simulink model "simulation_staticParameters"  (R2016b)
settings: Solver=VariableStepAuto  StartTime=0.0  StopTime=10  RelTol=1e-3
settings Model: Creator=user  LastModifiedBy=user

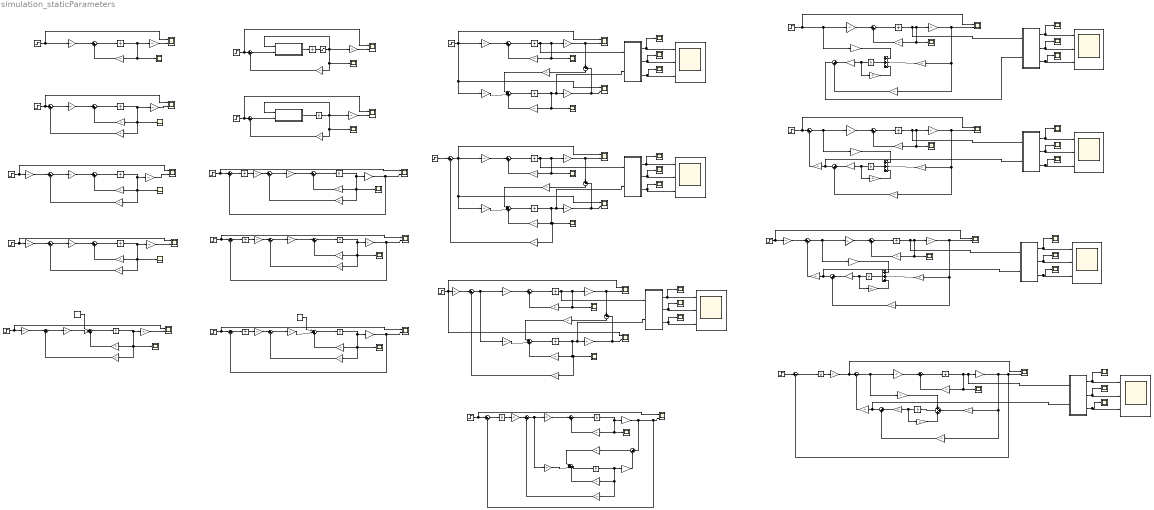
== system simulation_staticParameters ==
  note: FULL ORDER OBSERVER
  note: e_dot
  note: e
  note: y
  note: STATE FEEDBACK APPLIED
  note: NO STATE FEEDBACK
  note: input
  note: y
  note: x
  note: x_dot
  note: input
  note: y
  note: x
  note: x_dot
  note: STATE FEEDBACK + STATIC PRE-FILTER APPLIED
  note: input
  note: y
  note: x
  note: x_dot
  note: STATE FEEDBACK + STATIC PRE-FILTER APPLIED: PARAMETER CHANGE
  note: input
  note: y
  note: x
  note: x_dot
  note: STATE FEEDBACK + STATIC PRE-FILTER APPLIED: CONST DISTURBANCE
  note: input
  note: y
  note: x
  note: x_dot
  note: STATE FEEDBACK APPLIED on NONLINEAR SYSTEM
  note: input
  note: y
  note: STATE FEEDBACK APPLIED on NONLINEAR SYSTEM: zero inititial conditions
  note: input
  note: y
  note: STATE FEEDBACK + DYNAMIC COMPENSATOR APPLIED
  note: input
  note: x
  note: x_dot
  note: y
  note: STATE FEEDBACK + DYNAMIC COMPENSATOR APPLIED : PARAMETER CHANGE
  note: input
  note: x
  note: x_dot
  note: STATE FEEDBACK + DYNAMIC COMPENSATOR APPLIED: CONST DISTURBANCE
  note: y
  note: input
  note: x
  note: x_dot
  note: input
  note: y
  note: x
  note: x_dot
  note: input
  note: y
  note: x
  note: x_dot
  note: STATE FEEDBACK USING FULL ORDER OBSERVER
  note: input
  note: y
  note: x
  note: x_dot
  note: input
  note: y
  note: x
  note: x_dot
  note: STATE FEEDBACK + STATIC PRE-FILTER USING FULL ORDER OBSERVER
  note: input
  note: y
  note: x
  note: x_dot
  note: input
  note: y
  note: x
  note: x_dot
  note: y
  note: STATE FEEDBACK + DYNAMIC COMPENSATOR USING FULL ORDER OBSERVER
  note: input
  note: x
  note: x_dot
  note: x
  note: x_dot
  note: x
  note: x_dot
  note: input
  note: y
  note: REDUCED ORDER OBSERVER
  note: x
  note: x_dot
  note: input
  note: y
  note: STATE FEEDBACK USING REDUCED ORDER OBSERVER
  note: x
  note: x_dot
  note: input
  note: y
  note: STATE FEEDBACK + STATIC PRE-FILTER USING REDUCED ORDER OBSERVER
  note: x
  note: x_dot
  note: input
  note: y
  note: STATE FEEDBACK + DYNAMIC COMPENSATOR USING REDUCED ORDER OBSERVER
  A{1..5,7..20} (19 alike) : Gain  Gain=[0,0.1963,0;-0.1963,0,0.9817;0,0,0]  Multiplication=Matrix(K*u)
  A6 : Gain  Gain=[0,0.1963,0;-0.1963,0,0.9817;0,0,0]*1.05  Multiplication=Matrix(K*u)
  B{,1..2,4,8..13} (10 alike) : Gain  Gain=[0.025, 0.025;0,0;-0.333, 0.333]  Multiplication=Matrix(K*u)
  B{5,7,14..15} (4 alike) : Gain  Gain=[0.025;0;-0.333]  Multiplication=Matrix(K*u)
  B3 : Gain  Gain=[0.025, 0.025;0,0;-0.333, 0.333]*1.2  Multiplication=Matrix(K*u)
  B6 : Gain  Gain=[0.025;0;-0.333]*1.1  Multiplication=Matrix(K*u)
  C{1..5,7,11..16,19..21} (15 alike) : Gain  Gain=[1,0,0;0,1,0]  Multiplication=Matrix(K*u)
  C{8,10,17..18} (4 alike) : Gain  Gain=[1,0,0;]  Multiplication=Matrix(K*u)
  C22 : Gain  Gain=[1,0,0]  Multiplication=Matrix(K*u)
  C6 : Gain  Gain=[1,0,0;0,1,0]*1.1  Multiplication=Matrix(K*u)
  C9 : Gain  Gain=[1,0,0;]*1.05  Multiplication=Matrix(K*u)
  Constant : Constant  Value=2
  Constant1 : Constant  Value=10
  D : Gain  Gain=-21
  D1 : Gain  Gain=-21
  D2 : Gain  Gain=-21
  D3 : Gain  Gain=[0 -470.63; 0.9817 -3.583]  Multiplication=Matrix(K*u)
  G^-1(0){,1..4} (5 alike) : Gain  Gain=[394.735, -188.5098; 406.3311, -94.8546]  Multiplication=Matrix(K*u)
  Gain1 : Gain  Gain=[-.308 .358]  Multiplication=Matrix(K*u)
  Gain2 : Gain  Gain=[-.308 .358]  Multiplication=Matrix(K*u)
  Gain3 : Gain  Gain=[388.4933, -184.5838, 31.2146; 395.0384, -90.9286, 56.4750]  Multiplication=Matrix(K*u)
  Gain4 : Gain  Gain=[388.4933, -184.5838, 31.2146; 395.0384, -90.9286, 56.4750]  Multiplication=Matrix(K*u)
  Gain5 : Gain  Gain=[-60.270750000000010;-0.456600000000000]  Multiplication=Matrix(K*u)
  Gain6 : Gain  Gain=[-71699, -18130, -5530]  Multiplication=Matrix(K*u)
  Integrator{,1..4,6..7,9,11,17..19,21} (13 alike) : Integrator  InitialCondition=[0,0,0]
  Integrator{8,10,12,20,30} (5 alike) : Integrator  InitialCondition=[0]
  Integrator{13,15,22,24,26,28} (6 alike) : Integrator  InitialCondition=[1,2,3]
  Integrator14 : Integrator  InitialCondition=[2,4,10]
  Integrator16 : Integrator  InitialCondition=[2,4,5]
  Integrator23 : Integrator  InitialCondition=4
  Integrator25 : Integrator  InitialCondition=4
  Integrator27 : Integrator
  Integrator29 : Integrator  InitialCondition=[4,5]
  Integrator5 : Integrator  InitialCondition=[0.05,0.01,0.1]
  K{,1..2,9..10,12} (6 alike) : Gain  Gain=[388.4933, -184.5838, 31.2146; 395.0384, -90.9286, 56.4750]  Multiplication=Matrix(K*u)
  K{6..8,11} (4 alike) : Gain  Gain=[-71699, -18130, -5530]  Multiplication=Matrix(K*u)
  K3 : Gain  Gain=[-2.324, -31.3649, -8.468; 19.532, -5.9637, 2.3224]  Multiplication=Matrix(K*u)
  K5 : Gain  Gain=[-2.324, -31.3649, -8.468; 19.532, -5.9637, 2.3224]  Multiplication=Matrix(K*u)
  Ki{,1..4} (5 alike) : Gain  Gain=[-209440]  Multiplication=Matrix(K*u)
  L : Gain  Gain=[21.998, 0.1916; -1.8526, 44.002; -37.5542, 492.0554]  Multiplication=Matrix(K*u)
  L1 : Gain  Gain=[21.998, 0.1916; -1.8526, 44.002; -37.5542, 492.0554]  Multiplication=Matrix(K*u)
  L2 : Gain  Gain=[21.998, 0.1916; -1.8526, 44.002; -37.5542, 492.0554]  Multiplication=Matrix(K*u)
  L3 : Gain  Gain=[66;7392;55141]  Multiplication=Matrix(K*u)
  MATLAB Function1 : MATLAB Function  TreatAsAtomicUnit=on
  MATLAB Function2 : MATLAB Function  TreatAsAtomicUnit=on
  MATLAB Function3 : MATLAB Function  TreatAsAtomicUnit=on
  MATLAB Function4 : MATLAB Function  TreatAsAtomicUnit=on
  MATLAB Function5 : MATLAB Function  TreatAsAtomicUnit=on
  MATLAB Function6 : MATLAB Function  TreatAsAtomicUnit=on
  MATLAB Function7 : MATLAB Function  TreatAsAtomicUnit=on
  R : Gain  Gain=[-.308 .358]  Multiplication=Matrix(K*u)
  Saturation : Saturate  UpperLimit=20  LowerLimit=-20
  Scope{,2,4,6,8,10,12..13,15,17,19,21,23,25,27,29,31,33,36,38,40} (21 alike) : Scope  NumInputPorts=2
  Scope{1,3,5,7,9,11,14,16,18,20,22,24,26,28,30,32,34..35,37,39,41} (21 alike) : Scope
  Step{1..7} (7 alike) : Step  Time=[2,4]  Before=[0,0]  After=[1,-.3]  SampleTime=0
  Step{8..10,14} (4 alike) : Step  Time=[2]  Before=[0]  After=[1]  SampleTime=0
  Step11 : Step  Time=[2,3]  Before=[1,1.5]  After=[2,2.5]  SampleTime=0
  Step12 : Step  Time=[2,3]  Before=[1,1.5]  After=[2,2.5]  SampleTime=0
  Step13 : Step  Time=[2,4]  Before=[0.5,-0.5]  After=[1,-.2]  SampleTime=0
  Step15 : Step  Time=[2,3]  Before=[0.5,1]  After=[1,2]  SampleTime=0
  Step16 : Step  Time=[2,3]  Before=[0.5,1]  After=[1,2]  SampleTime=0
  Step17 : Step  Time=[2,3]  Before=[0.5,1]  After=[1,2]  SampleTime=0
  Step18 : Step  Time=[2]  Before=[0.5]  After=[1]  SampleTime=0
  Sum{,2..3,5,11,14,20,23,27,31,36,38..40,42,45,47,49} (18 alike) : Sum  Inputs=|++
  Sum{1,4,6,8..10,12..13,15..16,18..19,22,25..26,29..30,32..33,35,43,46,50..51} (24 alike) : Sum  Inputs=|+-
  Sum{7,17,21,24,28,34} (6 alike) : Sum  Inputs=|+++
  Sum37 : Sum  Inputs=+|++
  Sum41 : Sum  Inputs=+|++
  Sum44 : Sum  Inputs=+|++
  Sum48 : Sum  Inputs=+++
  T : Gain  Gain=[25.1991 -449.0244]  Multiplication=Matrix(K*u)
  T1 : Gain  Gain=[25.1991 -449.0244]  Multiplication=Matrix(K*u)
  T2 : Gain  Gain=[25.1991 -449.0244]  Multiplication=Matrix(K*u)
  T3 : Gain  Gain=[-8595.6;2288]  Multiplication=Matrix(K*u)
  X{1..21} (21 alike) : Scope
  all X{,1..6} (7 alike) : Scope  NumInputPorts=3
  b : Gain  Gain=[.025 .025;0 0;-.333 .333]  Multiplication=Matrix(K*u)
  b1 : Gain  Gain=[.025 .025;0 0;-.333 .333]  Multiplication=Matrix(K*u)
  b2 : Gain  Gain=[.025 .025;0 0;-.333 .333]  Multiplication=Matrix(K*u)
  b3 : Gain  Gain=[.025;0;-.333]  Multiplication=Matrix(K*u)
  f1 : Gain  Gain=[1 0;0 1;-1 21.3915]  Multiplication=Matrix(K*u)
  f2 : Gain  Gain=[0;0;1]  Multiplication=Matrix(K*u)
  f3 : Gain  Gain=[1 0;0 1;-1 21.3915]  Multiplication=Matrix(K*u)
  f4 : Gain  Gain=[0;0;1]  Multiplication=Matrix(K*u)
  f5 : Gain  Gain=[1 0;0 1;-1 21.3915]  Multiplication=Matrix(K*u)
  f6 : Gain  Gain=[0;0;1]  Multiplication=Matrix(K*u)
  f7 : Gain  Gain=[1;18.3;2397.5]  Multiplication=Matrix(K*u)
  f8 : Gain  Gain=[0 0;0 1;1 0]  Multiplication=Matrix(K*u)
  non-linear system1 : MATLAB Function  TreatAsAtomicUnit=on
  non-linear system2 : MATLAB Function  TreatAsAtomicUnit=on
  wires:
  Sum/1 -> Integrator/1
  Integrator/1 -> C3/1, A16/1, Scope1/1, K/1
  B/1 -> Sum/1
  A16/1 -> Sum/2
  Sum1/1 -> B/1
  K/1 -> Sum1/2
  Step7/1 -> Scope4/1, Sum1/1
  Sum2/1 -> Integrator1/1
  Integrator1/1 -> Scope3/1, A1/1, C1/1
  B1/1 -> Sum2/1
  A1/1 -> Sum2/2
  Step1/1 -> B1/1, Scope2/1
  C1/1 -> Scope2/2
  Sum3/1 -> Integrator2/1
  Integrator2/1 -> C5/1, K12/1, A2/1, Scope5/1
  B2/1 -> Sum3/1
  A2/1 -> Sum3/2
  Sum4/1 -> B2/1
  K12/1 -> Sum4/2
  Step2/1 -> Scope12/1, G^-1(0)/1
  G^-1(0)/1 -> Sum4/1
  Sum5/1 -> Integrator3/1
  Integrator3/1 -> C6/1, K1/1, A3/1, Scope9/1
  B3/1 -> Sum5/1
  A3/1 -> Sum5/2
  Sum6/1 -> B3/1
  K1/1 -> Sum6/2
  C6/1 -> Scope6/2
  Step3/1 -> G^-1(0)1/1, Scope6/1
  G^-1(0)1/1 -> Sum6/1
  Sum7/1 -> Integrator4/1
  Integrator4/1 -> C2/1, K2/1, A4/1, Scope11/1
  B4/1 -> Sum7/2
  A4/1 -> Sum7/3
  Sum8/1 -> B4/1
  K2/1 -> Sum8/2
  C2/1 -> Scope8/2
  Step4/1 -> G^-1(0)2/1, Scope8/1
  G^-1(0)2/1 -> Sum8/1
  Constant/1 -> Sum7/1
  non-linear system2/1(e_dot) -> Integrator5/1
  K5/1 -> Sum10/2
  Step5/1 -> Scope10/1, Sum10/1
  C7/1 -> Scope10/2
  Integrator5/1 -> non-linear system2/1(e), C7/1, K5/1, Scope7/1
  Sum10/1 -> non-linear system2/2(u)
  C3/1 -> Scope4/2
  C5/1 -> Scope12/2
  non-linear system1/1(e_dot) -> Integrator6/1
  K3/1 -> Sum9/2
  Step6/1 -> Scope13/1, Sum9/1
  C4/1 -> Scope13/2
  Integrator6/1 -> Saturation/1
  Sum9/1 -> non-linear system1/2(u)
  Saturation/1 -> C4/1, K3/1, Scope14/1, non-linear system1/1(e)
  Sum11/1 -> Integrator7/1
  Integrator7/1 -> C8/1, A5/1, Scope16/1, K6/1
  B5/1 -> Sum11/1
  A5/1 -> Sum11/2
  Sum12/1 -> B5/1
  K6/1 -> Sum12/2
  Step8/1 -> Sum13/1, Scope15/1
  Ki/1 -> Sum12/1
  C8/1 -> Sum13/2, Scope15/2
  Integrator8/1 -> Ki/1
  Sum13/1 -> Integrator8/1
  Sum14/1 -> Integrator9/1
  Integrator9/1 -> C9/1, A6/1, Scope18/1, K7/1
  B6/1 -> Sum14/1
  A6/1 -> Sum14/2
  Sum15/1 -> B6/1
  K7/1 -> Sum15/2
  Step9/1 -> Sum16/1, Scope17/1
  Ki1/1 -> Sum15/1
  C9/1 -> Sum16/2, Scope17/2
  Integrator10/1 -> Ki1/1
  Sum16/1 -> Integrator10/1
  Sum17/1 -> Integrator11/1
  Integrator11/1 -> C10/1, A7/1, Scope20/1, K8/1
  B7/1 -> Sum17/2
  A7/1 -> Sum17/3
  Sum18/1 -> B7/1
  K8/1 -> Sum18/2
  Step10/1 -> Sum19/1, Scope19/1
  Ki2/1 -> Sum18/1
  C10/1 -> Sum19/2, Scope19/2
  Integrator12/1 -> Ki2/1
  Sum19/1 -> Integrator12/1
  Constant1/1 -> Sum17/1
  Sum20/1 -> Integrator13/1
  Integrator13/1 -> C11/1, Scope22/1, A8/1, MATLAB Function3/1(x)
  B8/1 -> Sum20/1
  A8/1 -> Sum20/2
  C11/1 -> Sum22/1, Scope21/2
  Sum21/1 -> Integrator14/1
  Integrator14/1 -> MATLAB Function3/2(x_hat), C12/1, Scope24/1, A9/1
  B9/1 -> Sum21/2
  A9/1 -> Sum21/3
  Step11/1 -> B9/1, Scope23/1, B8/1, Scope21/1
  C12/1 -> Sum22/2, Scope23/2
  Sum22/1 -> L/1
  L/1 -> Sum21/1
  MATLAB Function3/1(x1) -> all X/1, X1/1
  MATLAB Function3/2(x2) -> all X/2, X2/1
  MATLAB Function3/3(x3) -> X3/1, all X/3
  Sum23/1 -> Integrator15/1
  Integrator15/1 -> C13/1, Scope26/1, A10/1, MATLAB Function1/1(x)
  B10/1 -> Sum23/1
  A10/1 -> Sum23/2
  C13/1 -> Sum25/1, Scope25/2
  Sum24/1 -> Integrator16/1
  Integrator16/1 -> MATLAB Function1/2(x_hat), C14/1, K9/1, Scope28/1, A11/1
  B11/1 -> Sum24/2
  A11/1 -> Sum24/3
  Sum26/1 -> B11/1, Scope27/1, B10/1, Scope25/1
  C14/1 -> Sum25/2, Scope27/2
  Sum25/1 -> L1/1
  L1/1 -> Sum24/1
  MATLAB Function1/1(x1) -> X4/1, all X1/1
  MATLAB Function1/2(x2) -> all X1/2, X5/1
  MATLAB Function1/3(x3) -> all X1/3, X6/1
  Step12/1 -> Sum26/1
  K9/1 -> Sum26/2
  Sum27/1 -> Integrator17/1
  Integrator17/1 -> C15/1, Scope30/1, A12/1, MATLAB Function2/1(x)
  B12/1 -> Sum27/1
  A12/1 -> Sum27/2
  C15/1 -> Sum29/1, Scope29/2
  Sum28/1 -> Integrator18/1
  Integrator18/1 -> MATLAB Function2/2(x_hat), C16/1, K10/1, Scope32/1, A13/1
  B13/1 -> Sum28/2
  A13/1 -> Sum28/3
  Sum30/1 -> B13/1, B12/1
  C16/1 -> Sum29/2, Scope31/2
  Sum29/1 -> L2/1
  L2/1 -> Sum28/1
  MATLAB Function2/1(x1) -> X7/1, all X2/1
  MATLAB Function2/2(x2) -> all X2/2, X8/1
  MATLAB Function2/3(x3) -> all X2/3, X9/1
  K10/1 -> Sum30/2
  Step13/1 -> Scope31/1, Scope29/1, G^-1(0)3/1
  G^-1(0)3/1 -> Sum30/1
  Sum31/1 -> Integrator19/1
  Integrator19/1 -> C17/1, Scope34/1, A14/1
  B14/1 -> Sum31/1
  A14/1 -> Sum31/2
  K11/1 -> Sum32/2
  Step14/1 -> Sum33/1, Scope33/1
  Ki3/1 -> Sum32/1
  Integrator20/1 -> Ki3/1
  Sum33/1 -> Integrator20/1
  Sum34/1 -> Integrator21/1
  Integrator21/1 -> C18/1, K11/1, A15/1
  B15/1 -> Sum34/2
  A15/1 -> Sum34/3
  Sum32/1 -> B15/1, B14/1
  C17/1 -> Sum35/1, Sum33/2, Scope33/2
  Sum35/1 -> L3/1
  L3/1 -> Sum34/1
  C18/1 -> Sum35/2
  b/1 -> Sum36/1
  Integrator22/1 -> MATLAB Function4/1(x), C19/1, A17/1, Scope35/1
  Sum36/1 -> Integrator22/1
  A17/1 -> Sum36/2
  Step15/1 -> b/1, R/1, Scope/1  "u(t)"
  C19/1 -> T/1, f1/1, Scope/2
  R/1 -> Sum37/1
  T/1 -> Sum37/2
  Sum37/1 -> Integrator23/1  "z_dot"
  D/1 -> Sum37/3
  Integrator23/1 -> f2/1, D/1  "Z"
  f2/1 -> Sum38/1
  f1/1 -> Sum38/2
  Sum38/1 -> MATLAB Function4/2(x_hat)  "x_hat"
  MATLAB Function4/1(x1) -> all X3/1, X10/1
  MATLAB Function4/2(x2) -> all X3/2, X11/1
  MATLAB Function4/3(x3) -> X12/1, all X3/3
  b1/1 -> Sum40/1
  Integrator24/1 -> MATLAB Function5/1(x), C20/1, A18/1, Scope37/1
  Sum40/1 -> Integrator24/1
  A18/1 -> Sum40/2
  Sum43/1 -> b1/1, Gain2/1  "u(t)"
  C20/1 -> T1/1, f3/1, Scope36/2
  Gain2/1 -> Sum41/1
  T1/1 -> Sum41/2
  Sum41/1 -> Integrator25/1  "z_dot"
  D1/1 -> Sum41/3
  Integrator25/1 -> f4/1, D1/1  "Z"
  f4/1 -> Sum42/1
  f3/1 -> Sum42/2
  Step16/1 -> Scope36/1, Sum43/1
  Sum42/1 -> MATLAB Function5/2(x_hat), Gain3/1  "x_hat"
  MATLAB Function5/1(x1) -> all X4/1, X13/1
  MATLAB Function5/2(x2) -> all X4/2, X14/1
  MATLAB Function5/3(x3) -> X15/1, all X4/3
  Gain3/1 -> Sum43/2
  b2/1 -> Sum39/1
  Integrator26/1 -> MATLAB Function6/1(x), C21/1, A19/1, Scope39/1
  Sum39/1 -> Integrator26/1
  A19/1 -> Sum39/2
  Sum46/1 -> b2/1, Gain1/1  "u(t)"
  C21/1 -> T2/1, f5/1, Scope38/2
  Gain1/1 -> Sum44/1
  T2/1 -> Sum44/2
  Sum44/1 -> Integrator27/1  "z_dot"
  D2/1 -> Sum44/3
  Integrator27/1 -> f6/1, D2/1  "Z"
  f6/1 -> Sum45/1
  f5/1 -> Sum45/2
  G^-1(0)4/1 -> Sum46/1
  Sum45/1 -> MATLAB Function6/2(x_hat), Gain4/1  "x_hat"
  MATLAB Function6/1(x1) -> all X5/1, X16/1
  MATLAB Function6/2(x2) -> all X5/2, X17/1
  MATLAB Function6/3(x3) -> X18/1, all X5/3
  Gain4/1 -> Sum46/2
  Step17/1 -> Scope38/1, G^-1(0)4/1
  b3/1 -> Sum47/1
  Integrator28/1 -> MATLAB Function7/1(x), C22/1, A20/1, Scope41/1
  Sum47/1 -> Integrator28/1
  A20/1 -> Sum47/2
  Sum50/1 -> b3/1, Gain5/1  "u(t)"
  C22/1 -> T3/1, f7/1, Sum51/2, Scope40/2
  Gain5/1 -> Sum48/1
  T3/1 -> Sum48/2
  Sum48/1 -> Integrator29/1  "z_dot"
  D3/1 -> Sum48/3
  Integrator29/1 -> f8/1, D3/1  "Z"
  f8/1 -> Sum49/1
  f7/1 -> Sum49/2
  Ki4/1 -> Scope40/1, Sum50/1
  Sum49/1 -> MATLAB Function7/2(x_hat), Gain6/1  "x_hat"
  MATLAB Function7/1(x1) -> all X6/1, X19/1
  MATLAB Function7/2(x2) -> all X6/2, X20/1
  MATLAB Function7/3(x3) -> X21/1, all X6/3
  Gain6/1 -> Sum50/2
  Integrator30/1 -> Ki4/1
  Sum51/1 -> Integrator30/1
  Step18/1 -> Sum51/1

== matlab function simulation_staticParameters/non-linear system1 ==
  data: e input; e_dot output; u input
function e_dot  = fcn(e,u)
e_dot = [0;0;0];
e_dot(1)=(0.1963-u(1))*e(2) + 0.9817*cos(e(3))+(u(2)-0.9817);
e_dot(2)=(u(1)-0.1963)*e(1) + 0.9817*sin(e(3));
e_dot(3)=u(1);

== matlab function simulation_staticParameters/non-linear system2 ==
  data: e input; e_dot output; u input
function e_dot  = fcn(e,u)
e_dot = [0;0;0];
e_dot(1)=(0.1963-u(1))*e(2) + 0.9817*cos(e(3))+(u(2)-0.9817);
e_dot(2)=(u(1)-0.1963)*e(1) + 0.9817*sin(e(3));
e_dot(3)=u(1);

== matlab function simulation_staticParameters/MATLAB Function1 ==
  data: x input; x_hat input; x1 output; x2 output; x3 output
function [x1,x2,x3] = CP(x,x_hat)

x1=[x(1),x_hat(1)];
x2=[x(2),x_hat(2)];
x3=[x(3),x_hat(3)];

== matlab function simulation_staticParameters/MATLAB Function3 ==
  data: x input; x_hat input; x1 output; x2 output; x3 output
function [x1,x2,x3] = CP(x,x_hat)

x1=[x(1),x_hat(1)];
x2=[x(2),x_hat(2)];
x3=[x(3),x_hat(3)];

== matlab function simulation_staticParameters/MATLAB Function2 ==
  data: x input; x_hat input; x1 output; x2 output; x3 output
function [x1,x2,x3] = CP(x,x_hat)

x1=[x(1),x_hat(1)];
x2=[x(2),x_hat(2)];
x3=[x(3),x_hat(3)];

== matlab function simulation_staticParameters/MATLAB Function4 ==
  data: x input; x_hat input; x1 output; x2 output; x3 output
function [x1,x2,x3] = CP(x,x_hat)

x1=[x(1),x_hat(1)];
x2=[x(2),x_hat(2)];
x3=[x(3),x_hat(3)];

== matlab function simulation_staticParameters/MATLAB Function5 ==
  data: x input; x_hat input; x1 output; x2 output; x3 output
function [x1,x2,x3] = CP(x,x_hat)

x1=[x(1),x_hat(1)];
x2=[x(2),x_hat(2)];
x3=[x(3),x_hat(3)];

== matlab function simulation_staticParameters/MATLAB Function6 ==
  data: x input; x_hat input; x1 output; x2 output; x3 output
function [x1,x2,x3] = CP(x,x_hat)

x1=[x(1),x_hat(1)];
x2=[x(2),x_hat(2)];
x3=[x(3),x_hat(3)];

== matlab function simulation_staticParameters/MATLAB Function7 ==
  data: x input; x_hat input; x1 output; x2 output; x3 output
function [x1,x2,x3] = CP(x,x_hat)

x1=[x(1),x_hat(1)];
x2=[x(2),x_hat(2)];
x3=[x(3),x_hat(3)];
